simulink model "DEM_testbench_DACerrors_9lev"  (Simulink 8.1)
settings: Solver=FixedStepDiscrete  StartTime=0.0  StopTime=60e-3  RelTol=1e-3
values from neighbouring files (symbols this model uses):
  dem_dcin = 1    [init_DAC_3ele.m]    (also in init_DAC_8ele.m)
  dem_select = 4    [init_DAC_3ele.m]    (also in init_DAC_8ele.m)
  dem_sinamp = 2    [init_DAC_3ele.m]    (also in init_DAC_8ele.m = 7)
  dem_sinfreq = 4882.8125    [init_DAC_3ele.m]    (also in init_DAC_8ele.m)
undefined symbols (not defined in the file or in its folder): DACctrl, Fs
libraries: dspsigops x12, simulink x8, dspsrcs4 x2
settings Model: Creator=amyles  LastModifiedBy=amyles
settings DataIOCC: MaxDataPoints=50000
settings DebuggingCC: StrictBusMsg=Warning
settings SFSimCC: SimParseCustomCode=off

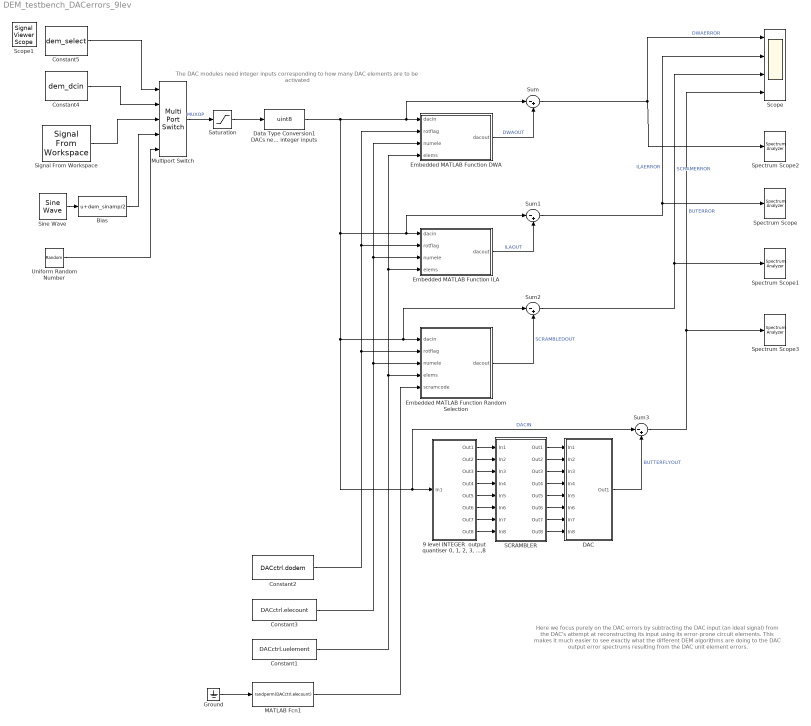
== system DEM_testbench_DACerrors_9lev ==
  note: The DAC modules need integer
      | inputs corresponding to how many
      | DAC elements are to be activated
  note: Here we focus purely on the DAC errors by
      | subtracting the DAC input (an ideal signal) from the
      | DAC's attempt at reconstructing its input using its
      | error-prone circuit elements.
      |
      | This makes it much easier to see exactly what the different
      | DEM algorithms are doing to the DAC output error
      | spectrums resulting from the DAC unit element errors.
  "9 level INTEGER  output quantiser 0, 1, 2, 3, ...,8" : Subsystem
  Bias : Bias  Bias=dem_sinamp/2
  Constant1 : Constant  Value=DACctrl.uelement  SampleTime=1/Fs
  Constant2 : Constant  Value=DACctrl.dodem  SampleTime=1/Fs
  Constant3 : Constant  Value=DACctrl.elecount  SampleTime=1/Fs
  Constant4 : Constant  Value=dem_dcin  SampleTime=1/Fs
  Constant5 : Constant  Value=dem_select  SampleTime=1/Fs
  DAC : Subsystem
  Data Type Conversion1 DACs need integer inputs : DataTypeConversion  OutDataTypeStr=uint8  RndMeth=Nearest
  Embedded MATLAB Function DWA : MATLAB Function  TreatAsAtomicUnit=on
  Embedded MATLAB Function ILA : MATLAB Function  TreatAsAtomicUnit=on
  Embedded MATLAB Function Random Selection : MATLAB Function  TreatAsAtomicUnit=on
  Ground : Ground
  MATLAB Fcn1 : MATLABFcn  MATLABFcn=randperm(DACctrl.elecount)  SampleTime=1/Fs
  Multiport Switch : MultiPortSwitch  Inputs=4
  SCRAMBLER : Subsystem
  Saturation : Saturate  UpperLimit=DACctrl.elecount  LowerLimit=0
  Scope : Scope  NumInputPorts=4
      settings: YMin=-0.04~-5~-5~-5  YMax=0.04~5~5~5
  Signal From Workspace : dspsrcs4/Signal From Workspace  X=[1 1 1 2]  Ts=1/Fs  nsamps=1  OutputAfterFinalValue=Cyclic repetition  ignoreOrWarnInputAndFrameLengths=off
  Sine Wave : dspsrcs4/Sine Wave  Amplitude=dem_sinamp/2  Frequency=dem_sinfreq  Phase=0  SampleMode=Discrete  OutComplex=Real  CompMethod=Trigonometric fcn  TableSize=Speed  SampleTime=1/Fs  SamplesPerFrame=1  ResetState=Restart at time zero  dataType=double  wordLen=16  udDataType=sfix(16)  fracBitsMode=Best precision  numFracBits=15  OutDataTypeStr=double  LastOutDataTypeStr=double
  Spectrum Scope{,1..3} (4 alike) : SpectrumAnalyzer
      settings: CopyFcn=scopeextensions.ScopeBlock.callback(gcbh, 'onBlockCopy', gcbh);  DeleteFcn=scopeextensions.ScopeBlock.callback(gcbh, 'onBlockDelete');  PreSaveFcn=scopeextensions.ScopeBlock.callback(gcbh, 'onModelSave');  NameChangeFcn=scopeextensions.ScopeBlock.callback(gcbh, 'onBlockRename');  CloseFcn=scopeextensions.ScopeBlock.callback(gcbh, 'onBlockClose');  PreDeleteFcn=scopeextensions.ScopeBlock.callback(gcbh, 'onBlockPreDelete');
  Sum{,1..3} (4 alike) : Sum  Inputs=|-+
  Uniform Random Number : UniformRandomNumber  Minimum=0  Maximum=DACctrl.elecount  SampleTime=1/Fs
  Scope1 : SignalViewerScope  IOType=viewer  NumInputPorts=2  ZoomMode=xonly  RefreshTime=0.035000
      settings: YMin=0~0  YMax=8~8
  wires:
  Constant5/1 -> Multiport Switch/1
  Signal From Workspace/1 -> Multiport Switch/3
  Sine Wave/1 -> Bias/1
  Multiport Switch/1 -> Saturation/1  "MUXOP"
  Data Type Conversion1 DACs need integer inputs/1 -> Embedded MATLAB Function ILA/1(dacin), Sum1/1, Embedded MATLAB Function Random Selection/1(dacin), Sum2/1, "9 level INTEGER  output quantiser 0, 1, 2, 3, ...,8"/1(In1), Sum3/1, Embedded MATLAB Function DWA/1(dacin), Sum/1  "DACIN"
  Saturation/1 -> Data Type Conversion1 DACs need integer inputs/1
  Bias/1 -> Multiport Switch/4
  Uniform Random Number/1 -> Multiport Switch/5
  Constant4/1 -> Multiport Switch/2
  Constant2/1 -> Embedded MATLAB Function DWA/2(rotflag), Embedded MATLAB Function ILA/2(rotflag), Embedded MATLAB Function Random Selection/2(rotflag)
  Constant3/1 -> Embedded MATLAB Function DWA/3(numele), Embedded MATLAB Function ILA/3(numele), Embedded MATLAB Function Random Selection/3(numele)
  Constant1/1 -> Embedded MATLAB Function DWA/4(elems), Embedded MATLAB Function ILA/4(elems), Embedded MATLAB Function Random Selection/4(elems)
  Embedded MATLAB Function DWA/1(dacout) -> Sum/2  "DWAOUT"
  Embedded MATLAB Function ILA/1(dacout) -> Sum1/2  "ILAOUT"
  Embedded MATLAB Function Random Selection/1(dacout) -> Sum2/2  "SCRAMBLEDOUT"
  Sum/1 -> Scope/1, Spectrum Scope2/1  "DWAERROR"
  Sum1/1 -> Scope/2, Spectrum Scope/1  "ILAERROR"
  Sum2/1 -> Spectrum Scope1/1, Scope/3  "SCRAMERROR"
  MATLAB Fcn1/1 -> Embedded MATLAB Function Random Selection/5(scramcode)
  Ground/1 -> MATLAB Fcn1/1
  "9 level INTEGER  output quantiser 0, 1, 2, 3, ...,8"/1(Out1) -> SCRAMBLER/1(In1)
  "9 level INTEGER  output quantiser 0, 1, 2, 3, ...,8"/2(Out2) -> SCRAMBLER/2(In2)
  "9 level INTEGER  output quantiser 0, 1, 2, 3, ...,8"/3(Out3) -> SCRAMBLER/3(In3)
  "9 level INTEGER  output quantiser 0, 1, 2, 3, ...,8"/4(Out4) -> SCRAMBLER/4(In4)
  "9 level INTEGER  output quantiser 0, 1, 2, 3, ...,8"/5(Out5) -> SCRAMBLER/5(In5)
  "9 level INTEGER  output quantiser 0, 1, 2, 3, ...,8"/6(Out6) -> SCRAMBLER/6(In6)
  "9 level INTEGER  output quantiser 0, 1, 2, 3, ...,8"/7(Out7) -> SCRAMBLER/7(In7)
  "9 level INTEGER  output quantiser 0, 1, 2, 3, ...,8"/8(Out8) -> SCRAMBLER/8(In8)
  SCRAMBLER/1(Out1) -> DAC/1(In1)
  SCRAMBLER/2(Out2) -> DAC/2(In2)
  SCRAMBLER/3(Out3) -> DAC/3(In3)
  SCRAMBLER/4(Out4) -> DAC/4(In4)
  SCRAMBLER/5(Out5) -> DAC/5(In5)
  SCRAMBLER/6(Out6) -> DAC/6(In6)
  SCRAMBLER/7(Out7) -> DAC/7(In7)
  SCRAMBLER/8(Out8) -> DAC/8(In8)
  DAC/1(Out1) -> Sum3/2  "BUTTERFLYOUT"
  Sum3/1 -> Spectrum Scope3/1, Scope/4  "BUTERROR"

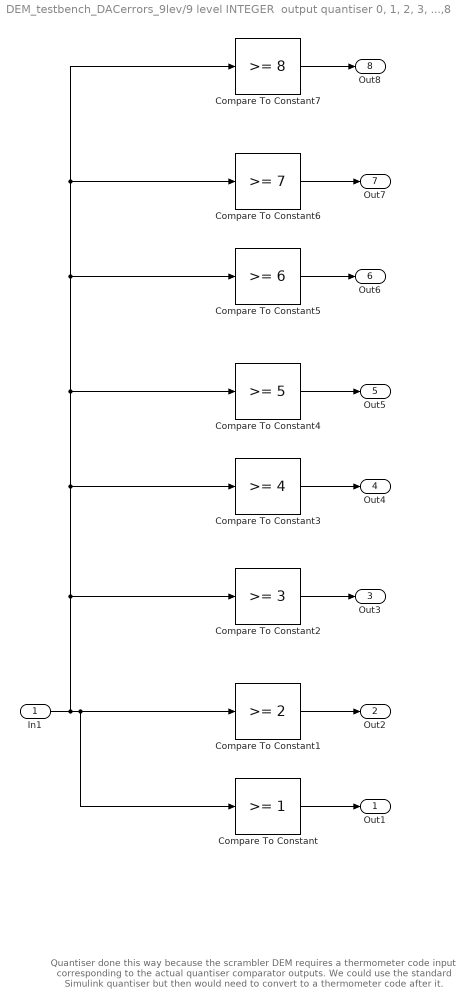
== system DEM_testbench_DACerrors_9lev/9 level INTEGER  output quantiser 0, 1, 2, 3, ...,8 ==
  note: Quantiser done this way because the scrambler DEM
      | requires a thermometer code input corresponding to
      | the actual quantiser comparator outputs. We could use the
      | standard Simulink quantiser but then would need to convert
      | to a thermometer code after it.
  In1 : Inport
  Compare To Constant : simulink/Logic and Bit Operations/Compare To Constant  SystemSampleTime=-1  relop=>=  const=1  LogicOutDataTypeMode=uint8
  Compare To Constant1 : simulink/Logic and Bit Operations/Compare To Constant  SystemSampleTime=-1  relop=>=  const=2  LogicOutDataTypeMode=uint8
  Compare To Constant2 : simulink/Logic and Bit Operations/Compare To Constant  SystemSampleTime=-1  relop=>=  const=3  LogicOutDataTypeMode=uint8
  Compare To Constant3 : simulink/Logic and Bit Operations/Compare To Constant  SystemSampleTime=-1  relop=>=  const=4  LogicOutDataTypeMode=uint8
  Compare To Constant4 : simulink/Logic and Bit Operations/Compare To Constant  SystemSampleTime=-1  relop=>=  const=5  LogicOutDataTypeMode=uint8
  Compare To Constant5 : simulink/Logic and Bit Operations/Compare To Constant  SystemSampleTime=-1  relop=>=  const=6  LogicOutDataTypeMode=uint8
  Compare To Constant6 : simulink/Logic and Bit Operations/Compare To Constant  SystemSampleTime=-1  relop=>=  const=7  LogicOutDataTypeMode=uint8
  Compare To Constant7 : simulink/Logic and Bit Operations/Compare To Constant  SystemSampleTime=-1  relop=>=  const=8  LogicOutDataTypeMode=uint8
  Out1 : Outport
  Out2 : Outport  Port=2
  Out3 : Outport  Port=3
  Out4 : Outport  Port=4
  Out5 : Outport  Port=5
  Out6 : Outport  Port=6
  Out7 : Outport  Port=7
  Out8 : Outport  Port=8
  wires:
  Compare To Constant2/1 -> Out3/1
  Compare To Constant1/1 -> Out2/1
  Compare To Constant/1 -> Out1/1
  In1/1 -> Compare To Constant1/1, Compare To Constant/1, Compare To Constant2/1, Compare To Constant3/1, Compare To Constant4/1, Compare To Constant5/1, Compare To Constant7/1, Compare To Constant6/1
  Compare To Constant5/1 -> Out6/1
  Compare To Constant4/1 -> Out5/1
  Compare To Constant3/1 -> Out4/1
  Compare To Constant7/1 -> Out8/1
  Compare To Constant6/1 -> Out7/1

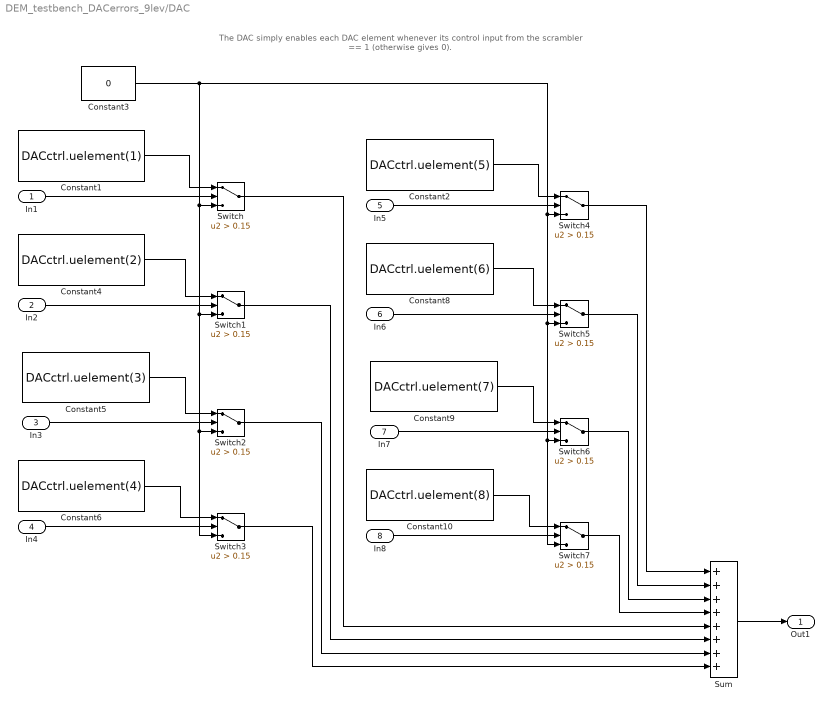
== system DEM_testbench_DACerrors_9lev/DAC ==
  note: The DAC simply enables each DAC element whenever its control
      | input from the scrambler == 1 (otherwise gives 0).
  In1 : Inport
  In2 : Inport  Port=2
  In3 : Inport  Port=3
  In4 : Inport  Port=4
  In5 : Inport  Port=5
  In6 : Inport  Port=6
  In7 : Inport  Port=7
  In8 : Inport  Port=8
  Constant1 : Constant  Value=DACctrl.uelement(1)  SampleTime=1/Fs
  Constant10 : Constant  Value=DACctrl.uelement(8)  SampleTime=1/Fs
  Constant2 : Constant  Value=DACctrl.uelement(5)  SampleTime=1/Fs
  Constant3 : Constant  Value=0  SampleTime=1/Fs
  Constant4 : Constant  Value=DACctrl.uelement(2)  SampleTime=1/Fs
  Constant5 : Constant  Value=DACctrl.uelement(3)  SampleTime=1/Fs
  Constant6 : Constant  Value=DACctrl.uelement(4)  SampleTime=1/Fs
  Constant8 : Constant  Value=DACctrl.uelement(6)  SampleTime=1/Fs
  Constant9 : Constant  Value=DACctrl.uelement(7)  SampleTime=1/Fs
  Sum : Sum  Inputs=++++++++
  Switch{,1..7} (8 alike) : Switch  Criteria=u2 > Threshold  Threshold=0.15
  Out1 : Outport
  wires:
  Constant6/1 -> Switch3/1
  Constant5/1 -> Switch2/1
  Constant4/1 -> Switch1/1
  Constant1/1 -> Switch/1
  Constant3/1 -> Switch3/3, Switch2/3, Switch1/3, Switch/3, Switch4/3, Switch5/3, Switch6/3, Switch7/3
  In4/1 -> Switch3/2
  In3/1 -> Switch2/2
  In2/1 -> Switch1/2
  In1/1 -> Switch/2
  Constant10/1 -> Switch7/1
  Constant9/1 -> Switch6/1
  Constant8/1 -> Switch5/1
  Constant2/1 -> Switch4/1
  In8/1 -> Switch7/2
  In7/1 -> Switch6/2
  In6/1 -> Switch5/2
  In5/1 -> Switch4/2
  Sum/1 -> Out1/1
  Switch4/1 -> Sum/1
  Switch5/1 -> Sum/2
  Switch6/1 -> Sum/3
  Switch7/1 -> Sum/4
  Switch/1 -> Sum/5
  Switch1/1 -> Sum/6
  Switch2/1 -> Sum/7
  Switch3/1 -> Sum/8

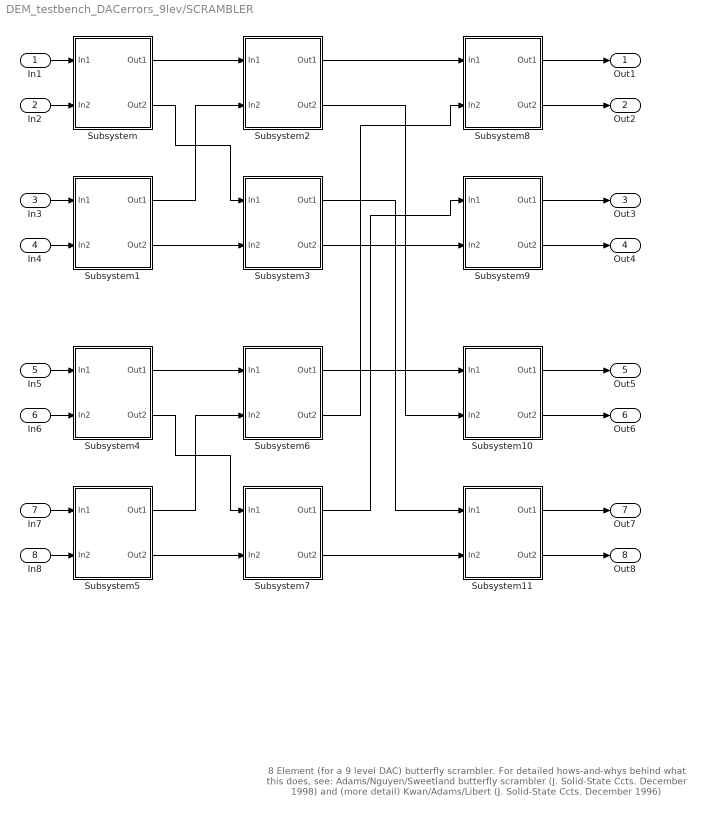
== system DEM_testbench_DACerrors_9lev/SCRAMBLER ==
  note: 8 Element (for a 9 level DAC) butterfly scrambler.
      |
      | For detailed hows-and-whys behind what this does, see:
      |
      | Adams/Nguyen/Sweetland butterfly scrambler
      | (J. Solid-State Ccts. December 1998)
      |
      | and (more detail)
      |
      | Kwan/Adams/Libert
      | (J. Solid-State Ccts. December 1996)
  In1 : Inport
  In2 : Inport  Port=2
  In3 : Inport  Port=3
  In4 : Inport  Port=4
  In5 : Inport  Port=5
  In6 : Inport  Port=6
  In7 : Inport  Port=7
  In8 : Inport  Port=8
  Subsystem : Subsystem
  Subsystem1 : Subsystem
  Subsystem10 : Subsystem
  Subsystem11 : Subsystem
  Subsystem2 : Subsystem
  Subsystem3 : Subsystem
  Subsystem4 : Subsystem
  Subsystem5 : Subsystem
  Subsystem6 : Subsystem
  Subsystem7 : Subsystem
  Subsystem8 : Subsystem
  Subsystem9 : Subsystem
  Out1 : Outport
  Out2 : Outport  Port=2
  Out3 : Outport  Port=3
  Out4 : Outport  Port=4
  Out5 : Outport  Port=5
  Out6 : Outport  Port=6
  Out7 : Outport  Port=7
  Out8 : Outport  Port=8
  wires:
  In4/1 -> Subsystem1/2(In2)
  In3/1 -> Subsystem1/1(In1)
  In2/1 -> Subsystem/2(In2)
  In1/1 -> Subsystem/1(In1)
  Subsystem/2(Out2) -> Subsystem3/1(In1)
  Subsystem1/1(Out1) -> Subsystem2/2(In2)
  Subsystem1/2(Out2) -> Subsystem3/2(In2)
  Subsystem/1(Out1) -> Subsystem2/1(In1)
  In8/1 -> Subsystem5/2(In2)
  In7/1 -> Subsystem5/1(In1)
  In6/1 -> Subsystem4/2(In2)
  In5/1 -> Subsystem4/1(In1)
  Subsystem4/2(Out2) -> Subsystem7/1(In1)
  Subsystem5/1(Out1) -> Subsystem6/2(In2)
  Subsystem5/2(Out2) -> Subsystem7/2(In2)
  Subsystem4/1(Out1) -> Subsystem6/1(In1)
  Subsystem6/1(Out1) -> Subsystem10/1(In1)
  Subsystem7/2(Out2) -> Subsystem11/2(In2)
  Subsystem2/1(Out1) -> Subsystem8/1(In1)
  Subsystem3/2(Out2) -> Subsystem9/2(In2)
  Subsystem3/1(Out1) -> Subsystem11/1(In1)
  Subsystem2/2(Out2) -> Subsystem10/2(In2)
  Subsystem6/2(Out2) -> Subsystem8/2(In2)
  Subsystem7/1(Out1) -> Subsystem9/1(In1)
  Subsystem8/1(Out1) -> Out1/1
  Subsystem8/2(Out2) -> Out2/1
  Subsystem9/1(Out1) -> Out3/1
  Subsystem9/2(Out2) -> Out4/1
  Subsystem10/1(Out1) -> Out5/1
  Subsystem10/2(Out2) -> Out6/1
  Subsystem11/1(Out1) -> Out7/1
  Subsystem11/2(Out2) -> Out8/1

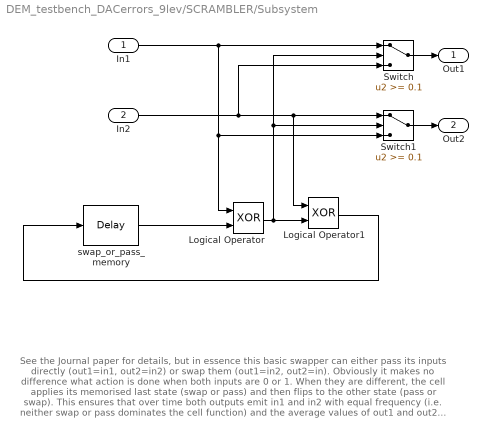
== system DEM_testbench_DACerrors_9lev/SCRAMBLER/Subsystem ==
  note: See the Journal paper for details, but in essence this basic swapper
      | can either pass its inputs directly (out1=in1, out2=in2) or swap
      | them (out1=in2, out2=in). Obviously it makes no difference what
      | action is done when both inputs are 0 or 1. When they are different,
      | the cell applies its memorised last state (swap or pass) and then flips
      | to the other state (pass or swap). This ensures that over time
      | both outputs emit in1 and in2 with equal frequency (i.e. neither
      | swap or pass dominates the cell function) and the average values
      | of out1 and out2 are both (in1+in2)/2.
  In1 : Inport
  In2 : Inport  Port=2
  Logical Operator : Logic  Operator=XOR  AllPortsSameDT=off  OutDataTypeStr=boolean
  Logical Operator1 : Logic  Operator=XOR  AllPortsSameDT=off  OutDataTypeStr=boolean
  Switch : Switch  Threshold=0.1
  Switch1 : Switch  Threshold=0.1
  swap_or_pass_memory : dspsigops/Delay  InputProcessing=Inherited (this choice will be removed - see release notes)  dly_unit=Samples  delay=1  ic_detail=off  dif_ic_for_ch=off  dif_ic_for_dly=off  ic=1  reset_popup=None
  Out1 : Outport
  Out2 : Outport  Port=2
  wires:
  Switch1/1 -> Out2/1
  Switch/1 -> Out1/1
  swap_or_pass_memory/1 -> Logical Operator/2
  Logical Operator1/1 -> swap_or_pass_memory/1
  Logical Operator/1 -> Logical Operator1/2, Switch1/2, Switch/2
  In2/1 -> Switch/3, Switch1/1, Logical Operator1/1
  In1/1 -> Switch/1, Switch1/3, Logical Operator/1

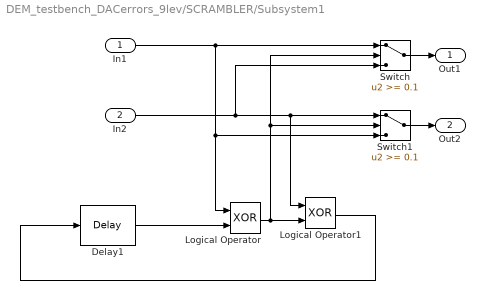
== system DEM_testbench_DACerrors_9lev/SCRAMBLER/Subsystem1 ==
  In1 : Inport
  In2 : Inport  Port=2
  Delay1 : dspsigops/Delay  dly_unit=Samples  delay=1  ic_detail=off  dif_ic_for_ch=off  dif_ic_for_dly=off  ic=0  reset_popup=None
  Logical Operator : Logic  Operator=XOR  AllPortsSameDT=off  OutDataTypeStr=boolean
  Logical Operator1 : Logic  Operator=XOR  AllPortsSameDT=off  OutDataTypeStr=boolean
  Switch : Switch  Threshold=0.1
  Switch1 : Switch  Threshold=0.1
  Out1 : Outport
  Out2 : Outport  Port=2
  wires:
  In1/1 -> Logical Operator/1, Switch1/3, Switch/1
  In2/1 -> Logical Operator1/1, Switch1/1, Switch/3
  Logical Operator/1 -> Switch/2, Switch1/2, Logical Operator1/2
  Logical Operator1/1 -> Delay1/1
  Delay1/1 -> Logical Operator/2
  Switch/1 -> Out1/1
  Switch1/1 -> Out2/1

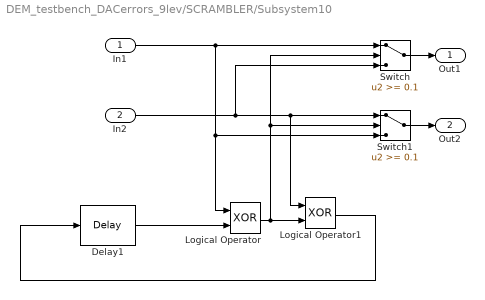
== system DEM_testbench_DACerrors_9lev/SCRAMBLER/Subsystem10 ==
  In1 : Inport
  In2 : Inport  Port=2
  Delay1 : dspsigops/Delay  dly_unit=Samples  delay=1  ic_detail=off  dif_ic_for_ch=off  dif_ic_for_dly=off  ic=0  reset_popup=None
  Logical Operator : Logic  Operator=XOR  AllPortsSameDT=off  OutDataTypeStr=boolean
  Logical Operator1 : Logic  Operator=XOR  AllPortsSameDT=off  OutDataTypeStr=boolean
  Switch : Switch  Threshold=0.1
  Switch1 : Switch  Threshold=0.1
  Out1 : Outport
  Out2 : Outport  Port=2
  wires:
  In1/1 -> Logical Operator/1, Switch1/3, Switch/1
  In2/1 -> Logical Operator1/1, Switch1/1, Switch/3
  Logical Operator/1 -> Switch/2, Switch1/2, Logical Operator1/2
  Logical Operator1/1 -> Delay1/1
  Delay1/1 -> Logical Operator/2
  Switch/1 -> Out1/1
  Switch1/1 -> Out2/1

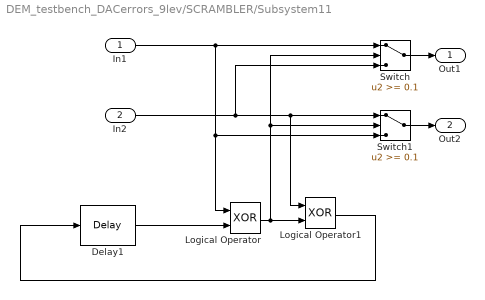
== system DEM_testbench_DACerrors_9lev/SCRAMBLER/Subsystem11 ==
  In1 : Inport
  In2 : Inport  Port=2
  Delay1 : dspsigops/Delay  dly_unit=Samples  delay=1  ic_detail=off  dif_ic_for_ch=off  dif_ic_for_dly=off  ic=0  reset_popup=None
  Logical Operator : Logic  Operator=XOR  AllPortsSameDT=off  OutDataTypeStr=boolean
  Logical Operator1 : Logic  Operator=XOR  AllPortsSameDT=off  OutDataTypeStr=boolean
  Switch : Switch  Threshold=0.1
  Switch1 : Switch  Threshold=0.1
  Out1 : Outport
  Out2 : Outport  Port=2
  wires:
  Switch1/1 -> Out2/1
  Switch/1 -> Out1/1
  Delay1/1 -> Logical Operator/2
  Logical Operator1/1 -> Delay1/1
  Logical Operator/1 -> Logical Operator1/2, Switch1/2, Switch/2
  In2/1 -> Switch/3, Switch1/1, Logical Operator1/1
  In1/1 -> Switch/1, Switch1/3, Logical Operator/1

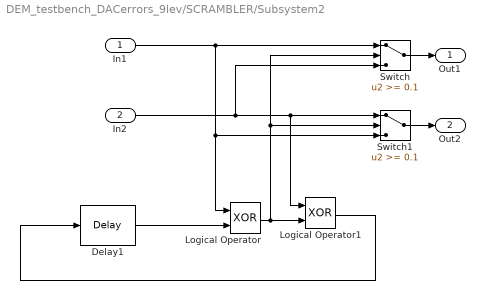
== system DEM_testbench_DACerrors_9lev/SCRAMBLER/Subsystem2 ==
  In1 : Inport
  In2 : Inport  Port=2
  Delay1 : dspsigops/Delay  dly_unit=Samples  delay=1  ic_detail=off  dif_ic_for_ch=off  dif_ic_for_dly=off  ic=0  reset_popup=None
  Logical Operator : Logic  Operator=XOR  AllPortsSameDT=off  OutDataTypeStr=boolean
  Logical Operator1 : Logic  Operator=XOR  AllPortsSameDT=off  OutDataTypeStr=boolean
  Switch : Switch  Threshold=0.1
  Switch1 : Switch  Threshold=0.1
  Out1 : Outport
  Out2 : Outport  Port=2
  wires:
  In1/1 -> Logical Operator/1, Switch1/3, Switch/1
  In2/1 -> Logical Operator1/1, Switch1/1, Switch/3
  Logical Operator/1 -> Switch/2, Switch1/2, Logical Operator1/2
  Logical Operator1/1 -> Delay1/1
  Delay1/1 -> Logical Operator/2
  Switch/1 -> Out1/1
  Switch1/1 -> Out2/1

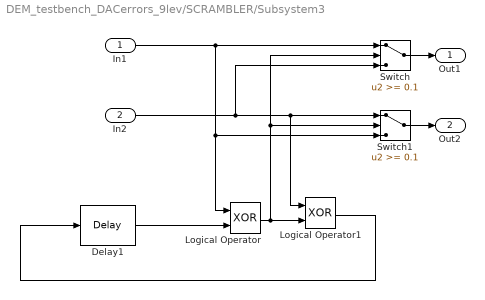
== system DEM_testbench_DACerrors_9lev/SCRAMBLER/Subsystem3 ==
  In1 : Inport
  In2 : Inport  Port=2
  Delay1 : dspsigops/Delay  dly_unit=Samples  delay=1  ic_detail=off  dif_ic_for_ch=off  dif_ic_for_dly=off  ic=0  reset_popup=None
  Logical Operator : Logic  Operator=XOR  AllPortsSameDT=off  OutDataTypeStr=boolean
  Logical Operator1 : Logic  Operator=XOR  AllPortsSameDT=off  OutDataTypeStr=boolean
  Switch : Switch  Threshold=0.1
  Switch1 : Switch  Threshold=0.1
  Out1 : Outport
  Out2 : Outport  Port=2
  wires:
  Switch1/1 -> Out2/1
  Switch/1 -> Out1/1
  Delay1/1 -> Logical Operator/2
  Logical Operator1/1 -> Delay1/1
  Logical Operator/1 -> Logical Operator1/2, Switch1/2, Switch/2
  In2/1 -> Switch/3, Switch1/1, Logical Operator1/1
  In1/1 -> Switch/1, Switch1/3, Logical Operator/1

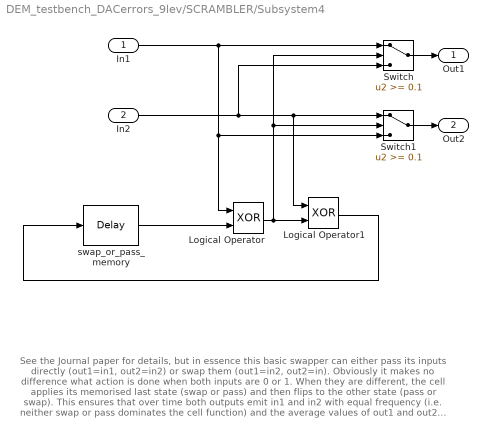
== system DEM_testbench_DACerrors_9lev/SCRAMBLER/Subsystem4 ==
  note: See the Journal paper for details, but in essence this basic swapper
      | can either pass its inputs directly (out1=in1, out2=in2) or swap
      | them (out1=in2, out2=in). Obviously it makes no difference what
      | action is done when both inputs are 0 or 1. When they are different,
      | the cell applies its memorised last state (swap or pass) and then flips
      | to the other state (pass or swap). This ensures that over time
      | both outputs emit in1 and in2 with equal frequency (i.e. neither
      | swap or pass dominates the cell function) and the average values
      | of out1 and out2 are both (in1+in2)/2.
  In1 : Inport
  In2 : Inport  Port=2
  Logical Operator : Logic  Operator=XOR  AllPortsSameDT=off  OutDataTypeStr=boolean
  Logical Operator1 : Logic  Operator=XOR  AllPortsSameDT=off  OutDataTypeStr=boolean
  Switch : Switch  Threshold=0.1
  Switch1 : Switch  Threshold=0.1
  swap_or_pass_memory : dspsigops/Delay  dly_unit=Samples  delay=1  ic_detail=off  dif_ic_for_ch=off  dif_ic_for_dly=off  ic=0  reset_popup=None
  Out1 : Outport
  Out2 : Outport  Port=2
  wires:
  In1/1 -> Logical Operator/1, Switch1/3, Switch/1
  In2/1 -> Logical Operator1/1, Switch1/1, Switch/3
  Logical Operator/1 -> Switch/2, Switch1/2, Logical Operator1/2
  Logical Operator1/1 -> swap_or_pass_memory/1
  swap_or_pass_memory/1 -> Logical Operator/2
  Switch/1 -> Out1/1
  Switch1/1 -> Out2/1

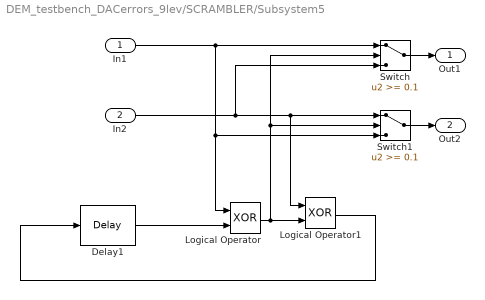
== system DEM_testbench_DACerrors_9lev/SCRAMBLER/Subsystem5 ==
  In1 : Inport
  In2 : Inport  Port=2
  Delay1 : dspsigops/Delay  dly_unit=Samples  delay=1  ic_detail=off  dif_ic_for_ch=off  dif_ic_for_dly=off  ic=0  reset_popup=None
  Logical Operator : Logic  Operator=XOR  AllPortsSameDT=off  OutDataTypeStr=boolean
  Logical Operator1 : Logic  Operator=XOR  AllPortsSameDT=off  OutDataTypeStr=boolean
  Switch : Switch  Threshold=0.1
  Switch1 : Switch  Threshold=0.1
  Out1 : Outport
  Out2 : Outport  Port=2
  wires:
  Switch1/1 -> Out2/1
  Switch/1 -> Out1/1
  Delay1/1 -> Logical Operator/2
  Logical Operator1/1 -> Delay1/1
  Logical Operator/1 -> Logical Operator1/2, Switch1/2, Switch/2
  In2/1 -> Switch/3, Switch1/1, Logical Operator1/1
  In1/1 -> Switch/1, Switch1/3, Logical Operator/1

== system DEM_testbench_DACerrors_9lev/SCRAMBLER/Subsystem6 ==
  In1 : Inport
  In2 : Inport  Port=2
  Delay1 : dspsigops/Delay  dly_unit=Samples  delay=1  ic_detail=off  dif_ic_for_ch=off  dif_ic_for_dly=off  ic=0  reset_popup=None
  Logical Operator : Logic  Operator=XOR  AllPortsSameDT=off  OutDataTypeStr=boolean
  Logical Operator1 : Logic  Operator=XOR  AllPortsSameDT=off  OutDataTypeStr=boolean
  Switch : Switch  Threshold=0.1
  Switch1 : Switch  Threshold=0.1
  Out1 : Outport
  Out2 : Outport  Port=2
  wires:
  Switch1/1 -> Out2/1
  Switch/1 -> Out1/1
  Delay1/1 -> Logical Operator/2
  Logical Operator1/1 -> Delay1/1
  Logical Operator/1 -> Logical Operator1/2, Switch1/2, Switch/2
  In2/1 -> Switch/3, Switch1/1, Logical Operator1/1
  In1/1 -> Switch/1, Switch1/3, Logical Operator/1

== system DEM_testbench_DACerrors_9lev/SCRAMBLER/Subsystem7 ==
  In1 : Inport
  In2 : Inport  Port=2
  Delay1 : dspsigops/Delay  dly_unit=Samples  delay=1  ic_detail=off  dif_ic_for_ch=off  dif_ic_for_dly=off  ic=0  reset_popup=None
  Logical Operator : Logic  Operator=XOR  AllPortsSameDT=off  OutDataTypeStr=boolean
  Logical Operator1 : Logic  Operator=XOR  AllPortsSameDT=off  OutDataTypeStr=boolean
  Switch : Switch  Threshold=0.1
  Switch1 : Switch  Threshold=0.1
  Out1 : Outport
  Out2 : Outport  Port=2
  wires:
  In1/1 -> Logical Operator/1, Switch1/3, Switch/1
  In2/1 -> Logical Operator1/1, Switch1/1, Switch/3
  Logical Operator/1 -> Switch/2, Switch1/2, Logical Operator1/2
  Logical Operator1/1 -> Delay1/1
  Delay1/1 -> Logical Operator/2
  Switch/1 -> Out1/1
  Switch1/1 -> Out2/1

== system DEM_testbench_DACerrors_9lev/SCRAMBLER/Subsystem8 ==
  In1 : Inport
  In2 : Inport  Port=2
  Delay1 : dspsigops/Delay  dly_unit=Samples  delay=1  ic_detail=off  dif_ic_for_ch=off  dif_ic_for_dly=off  ic=0  reset_popup=None
  Logical Operator : Logic  Operator=XOR  AllPortsSameDT=off  OutDataTypeStr=boolean
  Logical Operator1 : Logic  Operator=XOR  AllPortsSameDT=off  OutDataTypeStr=boolean
  Switch : Switch  Threshold=0.1
  Switch1 : Switch  Threshold=0.1
  Out1 : Outport
  Out2 : Outport  Port=2
  wires:
  Switch1/1 -> Out2/1
  Switch/1 -> Out1/1
  Delay1/1 -> Logical Operator/2
  Logical Operator1/1 -> Delay1/1
  Logical Operator/1 -> Logical Operator1/2, Switch1/2, Switch/2
  In2/1 -> Switch/3, Switch1/1, Logical Operator1/1
  In1/1 -> Switch/1, Switch1/3, Logical Operator/1

== system DEM_testbench_DACerrors_9lev/SCRAMBLER/Subsystem9 ==
  In1 : Inport
  In2 : Inport  Port=2
  Delay1 : dspsigops/Delay  dly_unit=Samples  delay=1  ic_detail=off  dif_ic_for_ch=off  dif_ic_for_dly=off  ic=0  reset_popup=None
  Logical Operator : Logic  Operator=XOR  AllPortsSameDT=off  OutDataTypeStr=boolean
  Logical Operator1 : Logic  Operator=XOR  AllPortsSameDT=off  OutDataTypeStr=boolean
  Switch : Switch  Threshold=0.1
  Switch1 : Switch  Threshold=0.1
  Out1 : Outport
  Out2 : Outport  Port=2
  wires:
  In1/1 -> Logical Operator/1, Switch1/3, Switch/1
  In2/1 -> Logical Operator1/1, Switch1/1, Switch/3
  Logical Operator/1 -> Switch/2, Switch1/2, Logical Operator1/2
  Logical Operator1/1 -> Delay1/1
  Delay1/1 -> Logical Operator/2
  Switch/1 -> Out1/1
  Switch1/1 -> Out2/1

== matlab function Embedded MATLAB Function ILA ==
  data: dacin input double; dacout output double; rotflag input double; numele input double; elems input double
function dacout = DAC(dacin, rotflag, numele, elems)
%#eml

% This function assumes a MATLAB workspace structures exists called
% DACctrl with contents:
%
% DACctrl.dodem = DEM enable flag, 0 = no ILA, 1 = apply ILA
% DACctrl.elecount = number fo unit elements in the DAC
% DACctrl.uelement(1) = size of first unit element
% ...
% DACctrl.uelement(elecount) = size of last unit element

% ------------------ Begin Copyright notice -----------------------------
%
% COPYRIGHT AND PROPERTY OF DIALOG SEMICONDUCTOR, 2012.
%
% THIS COPYRIGHT NOTICE MUST NOT BE REMOVED OR MODIFIED.
%
% Commerical use is not permitted.
%
% Installation on systems available for use in any way by commercial users
% is not permitted.
%
% Permission for use is granted by Dialog Semiconductor only for the
% purposes of teaching or studying course ELEE11080/PGEE11110 "Sigma
% Delta Data Converters" (or any renamed variant or descendant of
% this course) at the University of Edinburgh.
%
% Personal copying and/or modification is permitted only by students and
% teaching staff of course PGEE11110 solely for the purposes of delivering
% or studying course PGEE11110.
%
% All permissions for use of this or modified copies are revoked upon
% ceasation of teaching duties or completion or de-enrollment for any
% reason from course PGEE11110.
%
% ------------------- End Copyright notice ------------------------------

persistent ila_pointer; % Need a persistent rotator state

dacplus1 = dacin+1; % Quantiser starts at 0, MATLAB array indices at 1...

% static memory cannot be dynamic, so just allocate enough for
% any realistic DAC. Edit this function if you *really* need more
% than 100 DAC elements...

if isempty(ila_pointer)
    ila_pointer = ones(1,100);    % initialise per-code indices
end

if (rotflag == 0)
    ila_pointer(1,dacplus1) = 1;    % reset if not rotating
end

dacout = 0.0;
ipt = ila_pointer(1,dacplus1);
for indx = 1:1:dacin
    dacout = dacout + elems(ipt);
    ipt = mod(ipt, numele) + 1;
% Above line is a faster way of saying...
%     ila_pointer(dacplus1) = ila_pointer(dacplus1) + 1;
%     if (ila_pointer(dacplus1) > numele)
%         ila_pointer(dacplus1) = 1;
%    end
end
ila_pointer(1,dacplus1) = ipt;

end

== matlab function Embedded MATLAB Function DWA ==
  data: dacin input double; dacout output double; rotflag input double; numele input double; elems input double
function dacout = DAC(dacin, rotflag, numele, elems)
%#eml

% This function assumes a MATLAB workspace structures exists called
% DACctrl with contents:
%
% DACctrl.dodem = DEM enable flag, 0 = no DWA, 1 = apply DWA
% DACctrl.elecount = number fo unit elements in the DAC
% DACctrl.uelement(1) = size of first unit element
% ...
% DACctrl.uelement(elecount) = size of last unit element

% ------------------ Begin Copyright notice -----------------------------
%
% COPYRIGHT AND PROPERTY OF DIALOG SEMICONDUCTOR, 2012.
%
% THIS COPYRIGHT NOTICE MUST NOT BE REMOVED OR MODIFIED.
%
% Commerical use is not permitted.
%
% Installation on systems available for use in any way by commercial users
% is not permitted.
%
% Permission for use is granted by Dialog Semiconductor only for the
% purposes of teaching or studying course ELEE11080/PGEE11110 "Sigma
% Delta Data Converters" (or any renamed variant or descendant of
% this course) at the University of Edinburgh.
%
% Personal copying and/or modification is permitted only by students and
% teaching staff of course PGEE11110 solely for the purposes of delivering
% or studying course PGEE11110.
%
% All permissions for use of this or modified copies are revoked upon
% ceasation of teaching duties or completion or de-enrollment for any
% reason from course PGEE11110.
%
% ------------------- End Copyright notice ------------------------------

persistent dwa_pointer; % Need a persistent rotator state

if isempty(dwa_pointer) || (rotflag == 0)
    dwa_pointer = 1;    % initialise or reset if not rotating
end

dacout = 0.0;
for indx = 1:1:dacin
    dacout = dacout + elems(dwa_pointer);
    dwa_pointer = dwa_pointer + 1;
    if (dwa_pointer > numele)
        dwa_pointer = 1;
    end
end

end

== matlab function Embedded MATLAB Function Random Selection ==
  data: dacin input double; dacout output double; rotflag input double; numele input double; elems input double; scramcode input double
function dacout = DAC(dacin, rotflag, numele, elems, scramcode)
%#eml

% This function assumes a MATLAB workspace structures exists called
% DACctrl with contents:
%
% DACctrl.dodem = DEM enable flag, 0 = no scramble, 1 = scramble
% DACctrl.elecount = number fo unit elements in the DAC
% DACctrl.uelement(1) = size of first unit element
% ...
% DACctrl.uelement(elecount) = size of last unit element

%eml.extrinsic('randperm');

% This version allows dynamic resizing of the DAC by moving the randperm
% function call up a level... look how much slower that makes Simulink
% run though!

% ------------------ Begin Copyright notice -----------------------------
%
% COPYRIGHT AND PROPERTY OF DIALOG SEMICONDUCTOR, 2012.
%
% THIS COPYRIGHT NOTICE MUST NOT BE REMOVED OR MODIFIED.
%
% Commerical use is not permitted.
%
% Installation on systems available for use in any way by commercial users
% is not permitted.
%
% Permission for use is granted by Dialog Semiconductor only for the
% purposes of teaching or studying course ELEE11080/PGEE11110 "Sigma
% Delta Data Converters" (or any renamed variant or descendant of
% this course) at the University of Edinburgh.
%
% Personal copying and/or modification is permitted only by students and
% teaching staff of course PGEE11110 solely for the purposes of delivering
% or studying course PGEE11110.
%
% All permissions for use of this or modified copies are revoked upon
% ceasation of teaching duties or completion or de-enrollment for any
% reason from course PGEE11110.
%
% ------------------- End Copyright notice ------------------------------

if (rotflag == 0)
    dacout = sum(elems(1:dacin));
else
    dacout = sum(elems(scramcode(1:dacin)));
end

end
